simulink model "th_simulink"  (R2016a)
settings: Solver=FixedStepAuto  StartTime=0.0  StopTime=.5  FixedStep=.0001  RelTol=1e-3
settings Model: Creator=jhake  LastModifiedBy=jhake

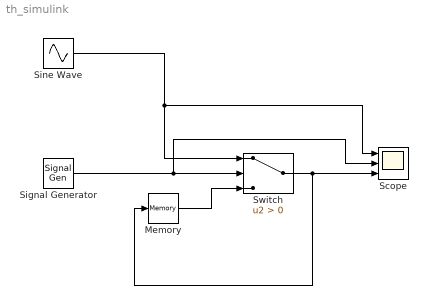
== system th_simulink ==
  Memory : Memory
  Scope : Scope  NumInputPorts=3
  Signal Generator : SignalGenerator  WaveForm=square  Frequency=100
  Sine Wave : Sin  Amplitude=.5  Bias=.5  Frequency=50  SampleTime=0
  Switch : Switch  Criteria=u2 > Threshold
  wires:
  Memory/1 -> Switch/3
  Sine Wave/1 -> Scope/1, Switch/1
  Signal Generator/1 -> Scope/2, Switch/2
  Switch/1 -> Memory/1, Scope/3
